simulink model "modelSPSid0"  (R2022a)
settings: Solver=ode45  StartTime=parSimulacio.ti  StopTime=0.1  MaxStep=parSimulacio.pas  RelTol=parSimulacio.tol  EnableMultiTasking=on
undefined symbols (not defined in the file or in its folder): parControl, parConvertidor, parGenerador, parMecanica, parSimulacio
libraries: simulink x7, spsMosfetLib x6, spsCurrentMeasurementLib x4, spsVoltageMeasurementLib x4, spsControlledCurrentSourceLib x3, spsDCVoltageSourceLib x2, spsSeriesRLCBranchLib x2, spspowerguiLib x1
settings Model: SimulationMode=accelerator  Creator=adria  LastModifiedBy=EEED Stores 381
settings SolverCC: AlgebraicLoopSolver=TrustRegion
settings DataIOCC: LimitDataPoints=on  SaveFormat=Array  SignalLoggingSaveFormat=ModelDataLogs  SaveOutput=off  SaveTime=off  ReturnWorkspaceOutputs=off
settings OptimizationCC: InitFltsAndDblsToZero=on  LifeSpan=inf
settings DebuggingCC: SaveWithParameterizedLinksMsg=none  UnderspecifiedInitializationDetection=Classic  MergeDetectMultiDrivingBlocksExec=none  SignalResolutionControl=TryResolveAllWithWarning  SolverPrmCheckMsg=warning  FcnCallInpInsideContextMsg=warning  UnconnectedInputMsg=warning  UnconnectedOutputMsg=warning  UnconnectedLineMsg=warning  SFUnexpectedBacktrackingDiag=warning  SFNoUnconditionalDefaultTransitionDiag=warning  SFExecutionAtInitializationDiag=none  SFMachineParentedDataDiag=warning  ArithmeticOperatorsInVariantConditions=warning
settings HardwareCC: ProdBitPerPointer=32  ProdBitPerSizeT=32  ProdBitPerPtrDiffT=32  ProdLargestAtomicFloat=None  ProdIntDivRoundTo=Undefined  ProdEndianess=Unspecified  ProdWordSize=32  ProdHWDeviceType=32-bit Generic
settings ModelReferenceCC: PropagateSignalLabelsOutOfModel=off
settings RTWCC: DLArmComputeVersion=19.05
settings CodeAppCC: StateflowObjectComments=on
settings GRTTargetCC: TargetFcnLib=ansi_tfl_tmw.mat  TargetLangStandard=C89/C90 (ANSI)  CombineOutputUpdateFcns=off  GRTInterface=on
settings ConfigComp: CovMetricSettings=dw  CovSaveCumulativeToWorkspaceVar=on  CovSaveSingleToWorkspaceVar=on

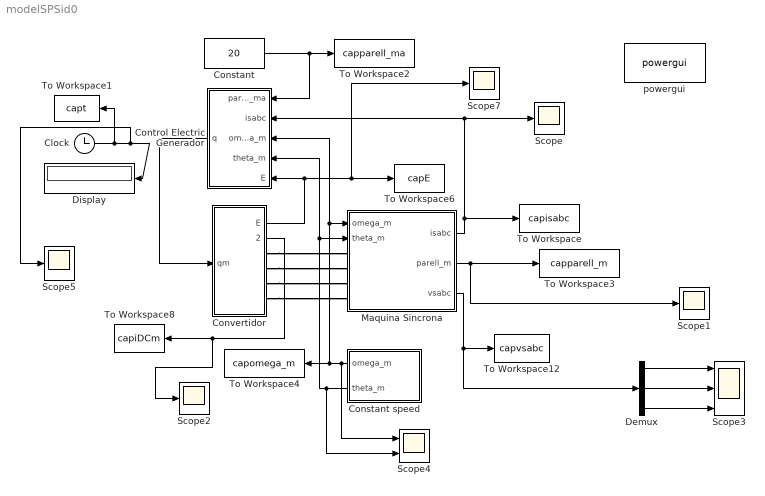
== system modelSPSid0 ==
  Clock : Clock
  Constant : Constant  Value=20
  Constant speed : Subsystem  mask{tempPar=parMecanica}
      mask prompts: tempPar "Estruc. Parametres"
      mask init:
      | omegat0=tempPar.omegat0;
  Control Electric Generador : Subsystem  mask{tempPar=parControl.Electric.Generador}
      mask prompts: tempPar "Estruc. Parametres"
      mask init:
      | rs=tempPar.rs;
      | Lq=tempPar.Lq;
      | Ld=tempPar.Ld;
      | lambda_m=tempPar.lambda_m;
      | P=tempPar.P;
      | %qKp=tempPar.qKp;
      | %qKi=tempPar.qKi;
      | %dKp=tempPar.dKp;
      | %dKi=tempPar.dKi;
      | dGcnum=tempPar.dGcnum;
      | dGcden=tempPar.dGcden;
      | qGcnum=tempPar.qGcnum;
      | qGcden=tempPar.qGcden;
      | T=tempPar.T;
      | SVPWM=tempPar.SVPWM;
  Convertidor : Subsystem  mask{tempPar=parConvertidor}
      mask prompts: tempPar "Estruc. Parametres"
      mask init:
      | E0=tempPar.E0;
      | C=tempPar.C;
  Demux : Demux  Outputs=3
  Display : Display
  Maquina Sincrona : Subsystem  mask{tempPar=parGenerador}
      mask prompts: tempPar "Estruct. Parametres"
      mask init:
      | rs=tempPar.rs;
      | Lq=tempPar.Lq;
      | Ld=tempPar.Ld;
      | lambda_m=tempPar.lambda_m;
      | P=tempPar.P;
      | isqd0=tempPar.isqd0;
  Scope{,1..2,5,7} (5 alike) : Scope
  Scope3 : Scope  NumInputPorts=3
  Scope4 : Scope  NumInputPorts=2
  To Workspace : ToWorkspace  VariableName=capisabc  SampleTime=parSimulacio.captura.Tmostreig
      settings: Decimation=parSimulacio.captura.Delmat
  To Workspace1 : ToWorkspace  VariableName=capt  SampleTime=parSimulacio.captura.Tmostreig
      settings: Decimation=parSimulacio.captura.Delmat
  To Workspace12 : ToWorkspace  VariableName=capvsabc  SampleTime=parSimulacio.captura.Tmostreig
      settings: Decimation=parSimulacio.captura.Delmat
  To Workspace2 : ToWorkspace  VariableName=capparell_ma  SampleTime=parSimulacio.captura.Tmostreig
      settings: Decimation=parSimulacio.captura.Delmat
  To Workspace3 : ToWorkspace  VariableName=capparell_m  SampleTime=parSimulacio.captura.Tmostreig
      settings: Decimation=parSimulacio.captura.Delmat
  To Workspace4 : ToWorkspace  VariableName=capomega_m  SampleTime=parSimulacio.captura.Tmostreig
      settings: Decimation=parSimulacio.captura.Delmat
  To Workspace6 : ToWorkspace  VariableName=capE  SampleTime=parSimulacio.captura.Tmostreig
      settings: Decimation=parSimulacio.captura.Delmat
  To Workspace8 : ToWorkspace  VariableName=capiDCm  SampleTime=parSimulacio.captura.Tmostreig
      settings: Decimation=parSimulacio.captura.Delmat
  powergui : spspowerguiLib/powergui  Priority=1  SimulationMode=Continuous  SampleTime=50e-6  frequency=60  Iterations=50  frequencyindice=0  Pbase=100e6  ErrMax=1e-4  UnitsV=kV  UnitsW=MW  buscounter=0  FunctionMessages=off  echomessages=off  EnableUseOfTLC=off  CurrentSourceSwitches=off  DisableSnubberDevices=off  DisableRonSwitches=off  DisableVfSwitches=off  DisplayEquations=off  AutomaticDiscreteSolvers=off  SolverType=Tustin/Backward Euler (TBE)  Interpol=off  ExternalGateDelay=off  methode=off  Ts=100  x0status=blocks  SPID=on  SwTol=0  HookPort=off  NonlinearTolerance=1e-4  nMaxIteration=100  ContinueOnMaxIteration=off  RestoreLinks=warning  ResistiveCurrentMeasurement=off  Frange=[0:2:500]  Ylog=off  Xlog=on  ShowGrid=off  save=off  variable=ZData  structure=0  ZoomFFT=off  StartTime=0.0  cycles=1  DisplayStyle=1  fundamental=60  FreqAxis=off  MaxFrequency=1000  frequencyindicesteady=1  RmsSteady=1  display=off
  wires:
  Clock/1 -> To Workspace1/1, Scope5/1, Display/1
  Control Electric Generador/1(q) -> Convertidor/1(qm)
  Convertidor/1(E) -> Control Electric Generador/5(E), Scope7/1, To Workspace6/1
  Convertidor/2(iDCm) -> Scope2/1, To Workspace8/1
  Maquina Sincrona/1(isabc) -> Control Electric Generador/2(isabc), Scope/1, To Workspace/1
  Maquina Sincrona/2(parell_m) -> Scope1/1, To Workspace3/1
  Constant speed/1(omega_m) -> Scope4/1, Maquina Sincrona/1(omega_m), Control Electric Generador/3(omega_m), To Workspace4/1
  Constant speed/2(theta_m) -> Scope4/2, Maquina Sincrona/2(theta_m), Control Electric Generador/4(theta_m)
  Maquina Sincrona/3(vsabc) -> To Workspace12/1, Demux/1
  Constant/1 -> Control Electric Generador/1(parell_ma), To Workspace2/1
  Demux/1 -> Scope3/1
  Demux/2 -> Scope3/2
  Demux/3 -> Scope3/3
  connections:
  Convertidor/RConn4 -- Maquina Sincrona/LConn4
  Convertidor/RConn3 -- Maquina Sincrona/LConn3
  Convertidor/RConn2 -- Maquina Sincrona/LConn2
  Convertidor/RConn1 -- Maquina Sincrona/LConn1

== system modelSPSid0/Constant speed ==
  Constant : Constant  Value=omegat0
  Constant1 : Constant  Value=pi/180
  Divide : Product  Inputs=*/  RndMeth=Zero  SaturateOnIntegerOverflow=on
  Divide1 : Product  Inputs=**  RndMeth=Zero  SaturateOnIntegerOverflow=on
  Integrator1 : Integrator
  Round : Rounding  Operator=round
  Scope : Scope  NumInputPorts=2
  Scope1 : Scope  NumInputPorts=2
  omega_m : Outport
  theta_m : Outport  Port=2
  wires:
  Constant/1 -> omega_m/1, Integrator1/1
  Integrator1/1 -> Scope/1, Divide/1
  Constant1/1 -> Divide1/2, Divide/2
  Divide/1 -> Scope1/1, Round/1
  Round/1 -> Scope1/2, Divide1/1
  Divide1/1 -> Scope/2, theta_m/1

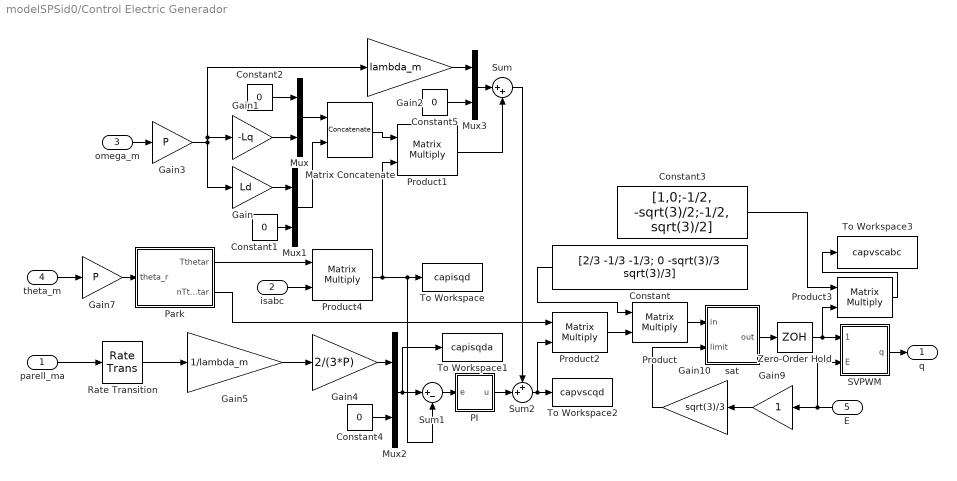
== system modelSPSid0/Control Electric Generador ==
  parell_ma : Inport
  isabc : Inport  Port=2  SampleTime=T
  omega_m : Inport  Port=3  SampleTime=T
  theta_m : Inport  Port=4  PortDimensions=1  SampleTime=T
  E : Inport  Port=5  SampleTime=T
  Constant : Constant  Value=[2/3 -1/3 -1/3; 0 -sqrt(3)/3 sqrt(3)/3]  SampleTime=T
  Constant{1..2,4..5} (4 alike) : Constant  Value=0  SampleTime=T
  Constant3 : Constant  Value=[1,0;-1/2, -sqrt(3)/2;-1/2, sqrt(3)/2]  SampleTime=T
  Gain : Gain  Gain=Ld
  Gain1 : Gain  Gain=-Lq
  Gain10 : Gain  Gain=sqrt(3)/3
  Gain2 : Gain  Gain=lambda_m
  Gain3 : Gain  Gain=P
  Gain4 : Gain  Gain=2/(3*P)
  Gain5 : Gain  Gain=1/lambda_m
  Gain7 : Gain  Gain=P
  Gain9 : Gain  SampleTime=T
  Matrix Concatenate : Concatenate  Mode=Multidimensional array  ConcatenateDimension=2
  Mux{,1..3} (4 alike) : Mux  Inputs=2
  PI : Subsystem
  Park : Subsystem
  Product{,1..4} (5 alike) : Product  Multiplication=Matrix(*)  RndMeth=Zero
  Rate Transition : RateTransition  OutPortSampleTime=T
  SVPWM : Subsystem  mask{TempPar=SVPWM}
      mask prompts: TempPar "Estructura de Parametres"
      mask init:
      | T=TempPar.T;
      | resolucio=TempPar.resolucio;
  Sum : Sum  Inputs=|++
  Sum1 : Sum  Inputs=|+-
  Sum2 : Sum  Inputs=++|
  To Workspace : ToWorkspace  VariableName=capisqd  SampleTime=parSimulacio.captura.Tmostreig
      settings: Decimation=parSimulacio.captura.Delmat
  To Workspace1 : ToWorkspace  VariableName=capisqda  SampleTime=parSimulacio.captura.Tmostreig
      settings: Decimation=parSimulacio.captura.Delmat
  To Workspace2 : ToWorkspace  VariableName=capvscqd  SampleTime=parSimulacio.captura.Tmostreig
      settings: Decimation=parSimulacio.captura.Delmat
  To Workspace3 : ToWorkspace  VariableName=capvscabc  SampleTime=parSimulacio.captura.Tmostreig
      settings: Decimation=parSimulacio.captura.Delmat
  Zero-Order Hold : ZeroOrderHold  SampleTime=T
  sat : Subsystem
  q : Outport
  wires:
  Gain7/1 -> Park/1(theta_r)
  Park/1(Tthetar) -> Product4/1
  Constant2/1 -> Mux/1
  Gain1/1 -> Mux/2
  Gain/1 -> Mux1/1
  Constant1/1 -> Mux1/2
  Mux/1 -> Matrix Concatenate/1
  Mux1/1 -> Matrix Concatenate/2
  Matrix Concatenate/1 -> Product1/1
  Product4/1 -> Product1/2, Sum1/2, To Workspace/1
  omega_m/1 -> Gain3/1
  Product1/1 -> Sum/2
  Sum2/1 -> Product2/2, To Workspace2/1
  Sum1/1 -> PI/1(e)
  PI/1(u) -> Sum2/2
  Mux2/1 -> Sum1/1, To Workspace1/1
  theta_m/1 -> Gain7/1
  isabc/1 -> Product4/2
  Gain3/1 -> Gain1/1, Gain2/1, Gain/1
  Mux3/1 -> Sum/1
  Gain2/1 -> Mux3/1
  Constant5/1 -> Mux3/2
  Park/2(nTthetar) -> Product2/1
  Sum/1 -> Sum2/1
  Gain4/1 -> Mux2/1
  Gain5/1 -> Gain4/1
  parell_ma/1 -> Rate Transition/1
  Rate Transition/1 -> Gain5/1
  Product/1 -> sat/1(in)
  sat/1(out) -> Zero-Order Hold/1
  Gain9/1 -> Gain10/1
  Gain10/1 -> sat/2(limit)
  Zero-Order Hold/1 -> SVPWM/1(valfbet), Product3/2
  E/1 -> Gain9/1, SVPWM/2(E)
  Product2/1 -> Product/2
  Constant/1 -> Product/1
  SVPWM/1(q) -> q/1
  Constant3/1 -> Product3/1
  Product3/1 -> To Workspace3/1
  Constant4/1 -> Mux2/2

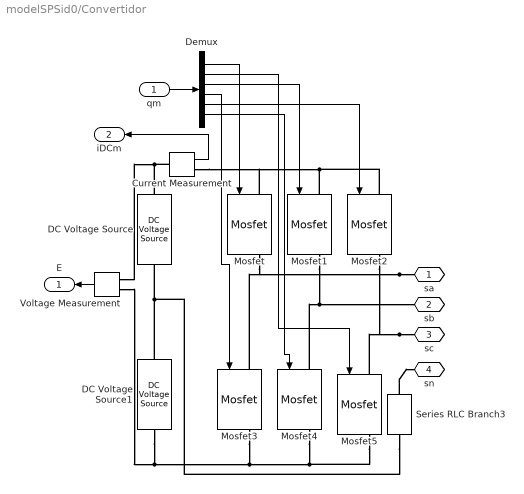
== system modelSPSid0/Convertidor ==
  qm : Inport
  Current Measurement : spsCurrentMeasurementLib/Current Measurement  PhasorSimulation=off  OutputType=Complex  PSBequivalent=0
  DC Voltage Source : spsDCVoltageSourceLib/DC Voltage Source  Amplitude=E0/2  Measurements=None
  DC Voltage Source1 : spsDCVoltageSourceLib/DC Voltage Source  Amplitude=E0/2  Measurements=None
  Demux : Demux  Outputs=6
  Mosfet{,1..5} (6 alike) : spsMosfetLib/Mosfet  Ron=0.1  Lon=0  Rd=0.01  Vfd=0  IC=0  Rs=1e5  Cs=inf  Measurements=on
  Series RLC Branch3 : spsSeriesRLCBranchLib/Series RLC Branch  LConnTagsString=__new0  RConnTagsString=__new0  BranchType=R  Resistance=1e5  Inductance=1e-3  SetiL0=off  InitialCurrent=0  Capacitance=1e-6  Setx0=off  InitialVoltage=0  Measurements=None
  Voltage Measurement : spsVoltageMeasurementLib/Voltage Measurement  PhasorSimulation=off  OutputType=Complex  PSBequivalent=0
  sa : PMIOPort  Side=Right
  sb : PMIOPort  Port=2  Side=Right
  sc : PMIOPort  Port=3  Side=Right
  sn : PMIOPort  Port=4  Side=Right
  E : Outport
  iDCm : Outport  Port=2
  wires:
  Voltage Measurement/1 -> E/1
  Demux/1 -> Mosfet/1
  Demux/3 -> Mosfet1/1
  Demux/5 -> Mosfet2/1
  Demux/2 -> Mosfet5/1
  Demux/4 -> Mosfet3/1
  Demux/6 -> Mosfet4/1
  qm/1 -> Demux/1
  Current Measurement/1 -> iDCm/1
  connections:
  sa/RConn1 -- Mosfet3/LConn1 -- Mosfet/RConn1
  Mosfet1/RConn1 -- Mosfet4/LConn1 -- sb/RConn1
  sc/RConn1 -- Mosfet5/LConn1 -- Mosfet2/RConn1
  Mosfet/LConn1 -- Current Measurement/RConn1 -- Mosfet2/LConn1 -- Mosfet1/LConn1
  Series RLC Branch3/RConn1 -- sn/RConn1
  DC Voltage Source1/RConn1 -- Series RLC Branch3/LConn1 -- DC Voltage Source/LConn1
  DC Voltage Source/RConn1 -- Voltage Measurement/LConn1 -- Current Measurement/LConn1
  DC Voltage Source1/LConn1 -- Voltage Measurement/LConn2 -- Mosfet3/RConn1 -- Mosfet5/RConn1 -- Mosfet4/RConn1

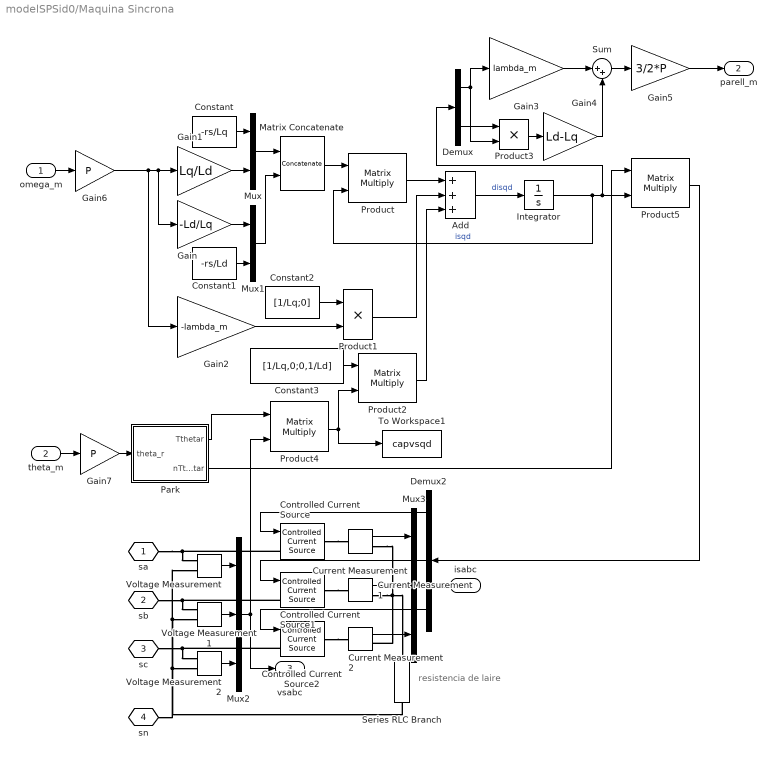
== system modelSPSid0/Maquina Sincrona ==
  note: resistencia
      | de laire
  omega_m : Inport
  theta_m : Inport  Port=2  PortDimensions=1
  Add : Sum  Inputs=+++
  Constant : Constant  Value=-rs/Lq
  Constant1 : Constant  Value=-rs/Ld
  Constant2 : Constant  Value=[1/Lq;0]
  Constant3 : Constant  Value=[1/Lq,0;0,1/Ld]
  Controlled Current Source : spsControlledCurrentSourceLib/Controlled Current Source  Initialize=on  Source_Type=AC  Amplitude=0  Phase=0  Frequency=0  Measurements=None
  Controlled Current Source1 : spsControlledCurrentSourceLib/Controlled Current Source  Initialize=on  Source_Type=AC  Amplitude=0  Phase=0  Frequency=0  Measurements=None
  Controlled Current Source2 : spsControlledCurrentSourceLib/Controlled Current Source  Initialize=on  Source_Type=AC  Amplitude=0  Phase=0  Frequency=0  Measurements=None
  Current Measurement : spsCurrentMeasurementLib/Current Measurement  PhasorSimulation=off  OutputType=Complex  PSBequivalent=0
  Current Measurement1 : spsCurrentMeasurementLib/Current Measurement  PhasorSimulation=off  OutputType=Complex  PSBequivalent=0
  Current Measurement2 : spsCurrentMeasurementLib/Current Measurement  PhasorSimulation=off  OutputType=Complex  PSBequivalent=0
  Demux : Demux  Outputs=2
  Demux2 : Demux  Outputs=3
  Gain : Gain  Gain=-Ld/Lq
  Gain1 : Gain  Gain=Lq/Ld
  Gain2 : Gain  Gain=-lambda_m
  Gain3 : Gain  Gain=lambda_m
  Gain4 : Gain  Gain=Ld-Lq
  Gain5 : Gain  Gain=3/2*P
  Gain6 : Gain  Gain=P
  Gain7 : Gain  Gain=P
  Integrator : Integrator  InitialCondition=isqd0
  Matrix Concatenate : Concatenate  Mode=Multidimensional array  ConcatenateDimension=2
  Mux : Mux  Inputs=2
  Mux1 : Mux  Inputs=2
  Mux2 : Mux  Inputs=3
  Mux3 : Mux  Inputs=3
  Park : Subsystem
  Product{,2,4..5} (4 alike) : Product  Multiplication=Matrix(*)  RndMeth=Zero
  Product1 : Product  RndMeth=Zero
  Product3 : Product  RndMeth=Zero
  Series RLC Branch : spsSeriesRLCBranchLib/Series RLC Branch  LConnTagsString=__new0  RConnTagsString=__new0  BranchType=R  Resistance=1e5  Inductance=1e-3  SetiL0=off  InitialCurrent=0  Capacitance=1e-6  Setx0=off  InitialVoltage=0  Measurements=None
  Sum : Sum  Inputs=|++
  To Workspace1 : ToWorkspace  VariableName=capvsqd  SampleTime=parSimulacio.captura.Tmostreig
      settings: Decimation=parSimulacio.captura.Delmat
  Voltage Measurement : spsVoltageMeasurementLib/Voltage Measurement  PhasorSimulation=off  OutputType=Complex  PSBequivalent=0
  Voltage Measurement1 : spsVoltageMeasurementLib/Voltage Measurement  PhasorSimulation=off  OutputType=Complex  PSBequivalent=0
  Voltage Measurement2 : spsVoltageMeasurementLib/Voltage Measurement  PhasorSimulation=off  OutputType=Complex  PSBequivalent=0
  sa : PMIOPort  Tag=PMCPort  Side=Left
  sb : PMIOPort  Tag=PMCPort  Port=2  Side=Left
  sc : PMIOPort  Tag=PMCPort  Port=3  Side=Left
  sn : PMIOPort  Tag=PMCPort  Port=4  Side=Left
  isabc : Outport
  parell_m : Outport  Port=2
  vsabc : Outport  Port=3
  wires:
  Constant/1 -> Mux/1
  Gain1/1 -> Mux/2
  Gain/1 -> Mux1/1
  Constant1/1 -> Mux1/2
  omega_m/1 -> Gain6/1
  Mux/1 -> Matrix Concatenate/1
  Mux1/1 -> Matrix Concatenate/2
  Matrix Concatenate/1 -> Product/1
  Product/1 -> Add/1
  Add/1 -> Integrator/1  "disqd"
  Integrator/1 -> Demux/1, Product5/2, Product/2  "isqd"
  Gain2/1 -> Product1/2
  Constant2/1 -> Product1/1
  Product1/1 -> Add/2
  Constant3/1 -> Product2/1
  Product2/1 -> Add/3
  Demux/1 -> Gain3/1, Product3/2
  Product3/1 -> Gain4/1
  Demux/2 -> Product3/1
  Gain3/1 -> Sum/1
  Gain4/1 -> Sum/2
  Sum/1 -> Gain5/1
  Gain5/1 -> parell_m/1
  Gain6/1 -> Gain1/1, Gain/1, Gain2/1
  theta_m/1 -> Gain7/1
  Product4/1 -> Product2/2, To Workspace1/1
  Park/1(Tthetar) -> Product4/1
  Gain7/1 -> Park/1(theta_r)
  Park/2(nTthetar) -> Product5/1
  Demux2/1 -> Controlled Current Source/1
  Demux2/2 -> Controlled Current Source1/1
  Demux2/3 -> Controlled Current Source2/1
  Voltage Measurement/1 -> Mux2/1
  Voltage Measurement1/1 -> Mux2/2
  Voltage Measurement2/1 -> Mux2/3
  Current Measurement/1 -> Mux3/1
  Current Measurement2/1 -> Mux3/3
  Product5/1 -> Demux2/1
  Current Measurement1/1 -> Mux3/2
  Mux3/1 -> isabc/1
  Mux2/1 -> Product4/2, vsabc/1
  connections:
  Controlled Current Source2/RConn1 -- Current Measurement2/LConn1
  Controlled Current Source1/RConn1 -- Current Measurement1/LConn1
  Controlled Current Source/RConn1 -- Current Measurement/LConn1
  Current Measurement/RConn1 -- Current Measurement2/RConn1 -- Current Measurement1/RConn1 -- Series RLC Branch/LConn1
  Controlled Current Source1/LConn1 -- Voltage Measurement1/LConn1 -- sb/RConn1
  Controlled Current Source2/LConn1 -- Voltage Measurement2/LConn1 -- sc/RConn1
  Controlled Current Source/LConn1 -- Voltage Measurement/LConn1 -- sa/RConn1
  sn/RConn1 -- Series RLC Branch/RConn1 -- Voltage Measurement2/LConn2 -- Voltage Measurement1/LConn2 -- Voltage Measurement/LConn2

== system modelSPSid0/Control Electric Generador/PI ==
  e : Inport
  Demux : Demux  Outputs=2
  Discrete Transfer Fcn : DiscreteTransferFcn  Numerator=[qGcnum]  Denominator=[qGcden]  SampleTime=T
  Discrete Transfer Fcn1 : DiscreteTransferFcn  Numerator=[dGcnum]  Denominator=[dGcden]  SampleTime=T
  Mux2 : Mux  Inputs=2
  u : Outport
  wires:
  Discrete Transfer Fcn/1 -> Mux2/1
  Discrete Transfer Fcn1/1 -> Mux2/2
  Demux/1 -> Discrete Transfer Fcn/1
  Demux/2 -> Discrete Transfer Fcn1/1
  e/1 -> Demux/1
  Mux2/1 -> u/1

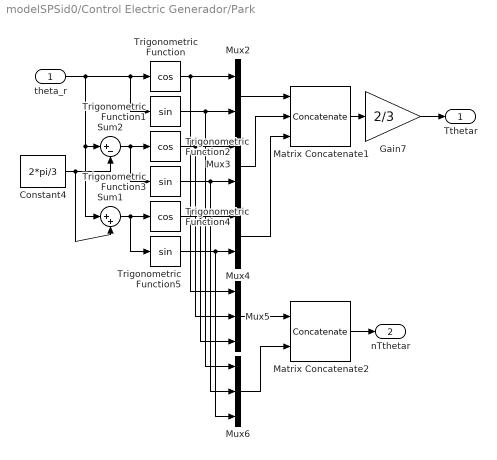
== system modelSPSid0/Control Electric Generador/Park ==
  theta_r : Inport
  Constant4 : Constant  Value=2*pi/3  SampleTime=T
  Gain7 : Gain  Gain=2/3
  Matrix Concatenate1 : Concatenate  NumInputs=3  Mode=Multidimensional array  ConcatenateDimension=2
  Matrix Concatenate2 : Concatenate  Mode=Multidimensional array  ConcatenateDimension=2
  Mux2 : Mux  Inputs=2
  Mux3 : Mux  Inputs=2
  Mux4 : Mux  Inputs=2
  Mux5 : Mux  Inputs=3
  Mux6 : Mux  Inputs=3
  Sum1 : Sum  Inputs=|++
  Sum2 : Sum  Inputs=|+-
  Trigonometric Function : Trigonometry  Operator=cos
  Trigonometric Function1 : Trigonometry
  Trigonometric Function2 : Trigonometry  Operator=cos
  Trigonometric Function3 : Trigonometry
  Trigonometric Function4 : Trigonometry  Operator=cos
  Trigonometric Function5 : Trigonometry
  Tthetar : Outport
  nTthetar : Outport  Port=2
  wires:
  theta_r/1 -> Sum1/1, Sum2/1, Trigonometric Function/1, Trigonometric Function1/1
  Sum2/1 -> Trigonometric Function2/1, Trigonometric Function3/1
  Sum1/1 -> Trigonometric Function4/1, Trigonometric Function5/1
  Constant4/1 -> Sum2/2, Sum1/2
  Trigonometric Function/1 -> Mux2/1, Mux5/1
  Trigonometric Function1/1 -> Mux2/2, Mux6/1
  Trigonometric Function2/1 -> Mux3/1, Mux5/2
  Trigonometric Function3/1 -> Mux3/2, Mux6/2
  Trigonometric Function4/1 -> Mux4/1, Mux5/3
  Trigonometric Function5/1 -> Mux4/2, Mux6/3
  Mux2/1 -> Matrix Concatenate1/1
  Mux3/1 -> Matrix Concatenate1/2
  Mux4/1 -> Matrix Concatenate1/3
  Matrix Concatenate1/1 -> Gain7/1
  Mux5/1 -> Matrix Concatenate2/1
  Mux6/1 -> Matrix Concatenate2/2
  Gain7/1 -> Tthetar/1
  Matrix Concatenate2/1 -> nTthetar/1

== system modelSPSid0/Control Electric Generador/SVPWM ==
  valfbet : Inport
  E : Inport  Port=2
  Calcul Periodes : Subsystem
  Dispars : Subsystem
  Divide1 : Product  Inputs=*/
  Gain1 : Gain  SampleTime=T
  Gain10 : Gain  Gain=sqrt(3)/3
  Mux : Mux  Inputs=6
  Rate Transition1 : RateTransition  OutPortSampleTime=T
  sat : Subsystem
  q : Outport
  wires:
  valfbet/1 -> Rate Transition1/1
  Calcul Periodes/1(t) -> Dispars/1(t)
  Calcul Periodes/2(n) -> Dispars/2(n)
  E/1 -> Gain1/1
  Rate Transition1/1 -> sat/1(in)
  Gain10/1 -> sat/2(limit)
  Divide1/1 -> Calcul Periodes/1(vsc)
  sat/1(out) -> Divide1/1
  Gain1/1 -> Gain10/1, Divide1/2
  Dispars/1(q1) -> Mux/1
  Dispars/2(q2) -> Mux/2
  Dispars/3(q3) -> Mux/3
  Dispars/4(q4) -> Mux/4
  Dispars/5(q5) -> Mux/5
  Dispars/6(q6) -> Mux/6
  Mux/1 -> q/1

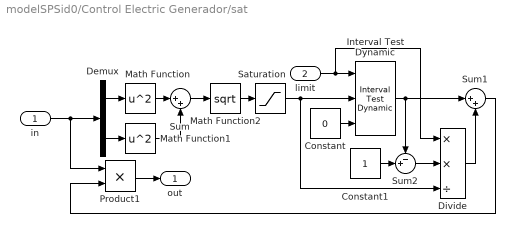
== system modelSPSid0/Control Electric Generador/sat ==
  in : Inport
  limit : Inport  Port=2
  Constant : Constant  Value=0  SampleTime=T
  Constant1 : Constant  SampleTime=T
  Demux : Demux  Outputs=2
  Divide : Product  Inputs=**/
  Interval Test Dynamic : simulink/Logic and Bit Operations/Interval Test Dynamic  IntervalClosedRight=on  IntervalClosedLeft=on  OutDataTypeStr=uint8
      settings: SourceProductBaseCode=SL
  Math Function : Math  Operator=square  SignedPower=on
  Math Function1 : Math  Operator=square  SignedPower=on
  Math Function2 : Math  Operator=sqrt  SignedPower=on
  Product1 : Product  RndMeth=Zero
  Saturation : Saturate  UpperLimit=inf  LowerLimit=1
  Sum : Sum  Inputs=|++
  Sum1 : Sum  Inputs=|++
  Sum2 : Sum  Inputs=-+|
  out : Outport
  wires:
  Math Function/1 -> Sum/1
  Math Function1/1 -> Sum/2
  Sum/1 -> Math Function2/1
  Math Function2/1 -> Saturation/1
  Demux/1 -> Math Function/1
  Demux/2 -> Math Function1/1
  in/1 -> Demux/1, Product1/1
  Product1/1 -> out/1
  Constant/1 -> Interval Test Dynamic/3
  Interval Test Dynamic/1 -> Sum1/1, Sum2/1
  Constant1/1 -> Sum2/2
  limit/1 -> Divide/1, Interval Test Dynamic/1
  Sum2/1 -> Divide/2
  Divide/1 -> Sum1/2
  Sum1/1 -> Product1/2
  Saturation/1 -> Divide/3, Interval Test Dynamic/2

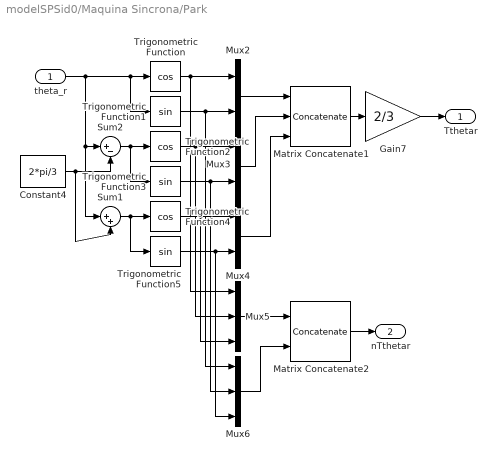
== system modelSPSid0/Maquina Sincrona/Park ==
  theta_r : Inport
  Constant4 : Constant  Value=2*pi/3
  Gain7 : Gain  Gain=2/3
  Matrix Concatenate1 : Concatenate  NumInputs=3  Mode=Multidimensional array  ConcatenateDimension=2
  Matrix Concatenate2 : Concatenate  Mode=Multidimensional array  ConcatenateDimension=2
  Mux2 : Mux  Inputs=2
  Mux3 : Mux  Inputs=2
  Mux4 : Mux  Inputs=2
  Mux5 : Mux  Inputs=3
  Mux6 : Mux  Inputs=3
  Sum1 : Sum  Inputs=|++
  Sum2 : Sum  Inputs=|+-
  Trigonometric Function : Trigonometry  Operator=cos
  Trigonometric Function1 : Trigonometry
  Trigonometric Function2 : Trigonometry  Operator=cos
  Trigonometric Function3 : Trigonometry
  Trigonometric Function4 : Trigonometry  Operator=cos
  Trigonometric Function5 : Trigonometry
  Tthetar : Outport
  nTthetar : Outport  Port=2
  wires:
  theta_r/1 -> Sum1/1, Sum2/1, Trigonometric Function/1, Trigonometric Function1/1
  Sum2/1 -> Trigonometric Function2/1, Trigonometric Function3/1
  Sum1/1 -> Trigonometric Function4/1, Trigonometric Function5/1
  Constant4/1 -> Sum2/2, Sum1/2
  Trigonometric Function/1 -> Mux2/1, Mux5/1
  Trigonometric Function1/1 -> Mux2/2, Mux6/1
  Trigonometric Function2/1 -> Mux3/1, Mux5/2
  Trigonometric Function3/1 -> Mux3/2, Mux6/2
  Trigonometric Function4/1 -> Mux4/1, Mux5/3
  Trigonometric Function5/1 -> Mux4/2, Mux6/3
  Mux2/1 -> Matrix Concatenate1/1
  Mux3/1 -> Matrix Concatenate1/2
  Mux4/1 -> Matrix Concatenate1/3
  Matrix Concatenate1/1 -> Gain7/1
  Mux5/1 -> Matrix Concatenate2/1
  Mux6/1 -> Matrix Concatenate2/2
  Gain7/1 -> Tthetar/1
  Matrix Concatenate2/1 -> nTthetar/1

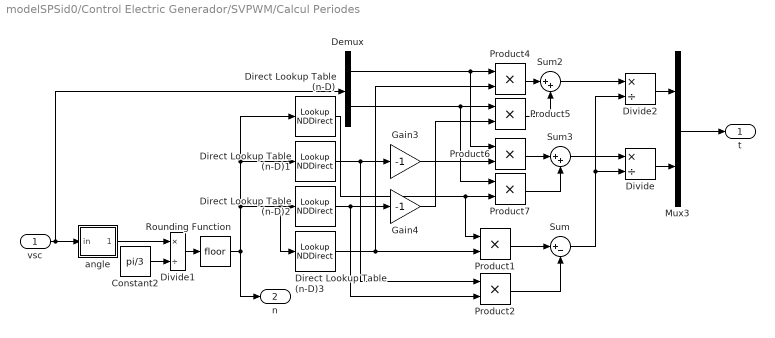
== system modelSPSid0/Control Electric Generador/SVPWM/Calcul Periodes ==
  vsc : Inport
  Constant2 : Constant  Value=pi/3  SampleTime=T
  Demux : Demux  Outputs=2
  Direct Lookup Table (n-D) : LookupNDDirect  NumberOfTableDimensions=1  Table=[2/3, 1/3, -1/3, -2/3, -1/3, 1/3]
  Direct Lookup Table (n-D)1 : LookupNDDirect  NumberOfTableDimensions=1  Table=[0, -sqrt(3)/3, -sqrt(3)/3, 0 ,sqrt(3)/3, sqrt(3)/3]
  Direct Lookup Table (n-D)2 : LookupNDDirect  NumberOfTableDimensions=1  Table=[1/3, -1/3, -2/3, -1/3, 1/3,2/3]
  Direct Lookup Table (n-D)3 : LookupNDDirect  NumberOfTableDimensions=1  Table=[-sqrt(3)/3, -sqrt(3)/3, 0 ,sqrt(3)/3, sqrt(3)/3,0]
  Divide : Product  Inputs=*/
  Divide1 : Product  Inputs=*/
  Divide2 : Product  Inputs=*/
  Gain3 : Gain  Gain=-1
  Gain4 : Gain  Gain=-1
  Mux3 : Mux  Inputs=2
  Product{1..2,4..7} (6 alike) : Product  RndMeth=Zero
  Rounding Function : Rounding
  Sum : Sum  Inputs=|+-
  Sum2 : Sum  Inputs=|++
  Sum3 : Sum  Inputs=|++
  angle : Subsystem
  t : Outport
  n : Outport  Port=2
  wires:
  angle/1(out) -> Divide1/1
  Constant2/1 -> Divide1/2
  Divide1/1 -> Rounding Function/1
  Rounding Function/1 -> n/1, Direct Lookup Table (n-D)1/1, Direct Lookup Table (n-D)/1, Direct Lookup Table (n-D)3/1, Direct Lookup Table (n-D)2/1
  vsc/1 -> angle/1(in), Demux/1
  Product1/1 -> Sum/1
  Product2/1 -> Sum/2
  Sum/1 -> Divide/2, Divide2/2
  Divide2/1 -> Mux3/1
  Divide/1 -> Mux3/2
  Mux3/1 -> t/1
  Product4/1 -> Sum2/1
  Product7/1 -> Sum3/2
  Sum3/1 -> Divide/1
  Sum2/1 -> Divide2/1
  Demux/1 -> Product4/1, Product6/1
  Demux/2 -> Product5/1, Product7/1
  Direct Lookup Table (n-D)3/1 -> Product4/2, Product1/2
  Direct Lookup Table (n-D)2/1 -> Product2/2, Gain4/1
  Gain4/1 -> Product5/2
  Direct Lookup Table (n-D)1/1 -> Gain3/1, Product2/1
  Gain3/1 -> Product6/2
  Direct Lookup Table (n-D)/1 -> Product7/2, Product1/1
  Product5/1 -> Sum2/2
  Product6/1 -> Sum3/1

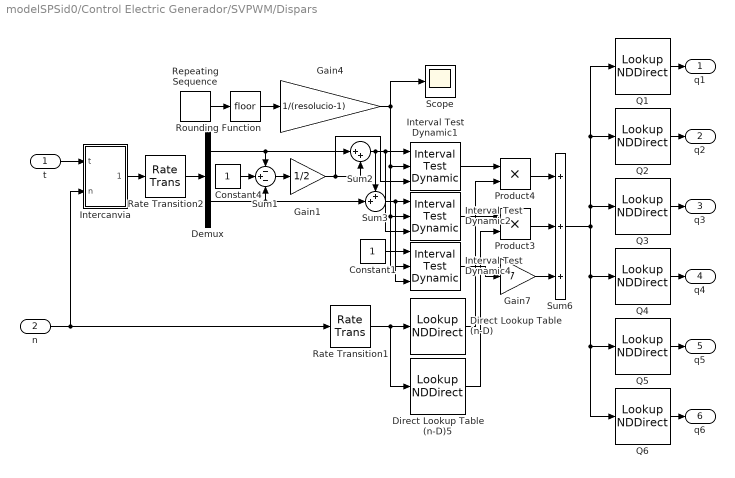
== system modelSPSid0/Control Electric Generador/SVPWM/Dispars ==
  t : Inport
  n : Inport  Port=2
  Constant1 : Constant  SampleTime=T/resolucio
  Constant4 : Constant  SampleTime=T/resolucio
  Demux : Demux  Outputs=2
  Direct Lookup Table (n-D) : LookupNDDirect  NumberOfTableDimensions=1  Table=[1,3,3,5,5,1]
  Direct Lookup Table (n-D)5 : LookupNDDirect  NumberOfTableDimensions=1  Table=[2,2,4,4,6,6]
  Gain1 : Gain  Gain=1/2  SampleTime=parControl.Electric.Generador.T/64
  Gain4 : Gain  Gain=1/(resolucio-1)  SampleTime=T/resolucio
  Gain7 : Gain  Gain=7
  Intercanvia : Subsystem
  Interval Test Dynamic1 : simulink/Logic and Bit Operations/Interval Test Dynamic  IntervalClosedRight=off  IntervalClosedLeft=on  OutDataTypeStr=uint8
      settings: SourceProductBaseCode=SL
  Interval Test Dynamic2 : simulink/Logic and Bit Operations/Interval Test Dynamic  IntervalClosedRight=off  IntervalClosedLeft=on  OutDataTypeStr=uint8
      settings: SourceProductBaseCode=SL
  Interval Test Dynamic4 : simulink/Logic and Bit Operations/Interval Test Dynamic  IntervalClosedRight=on  IntervalClosedLeft=on  OutDataTypeStr=uint8
      settings: SourceProductBaseCode=SL
  Product3 : Product  RndMeth=Zero
  Product4 : Product  RndMeth=Zero
  Q1 : LookupNDDirect  NumberOfTableDimensions=1  Table=[0,1,1,0,0,0,1,1]
  Q2 : LookupNDDirect  NumberOfTableDimensions=1  Table=[1,1,1,1,0,0,0,0]
  Q3 : LookupNDDirect  NumberOfTableDimensions=1  Table=[0,0,1,1,1,0,0,1]
  Q4 : LookupNDDirect  NumberOfTableDimensions=1  Table=[1,0,0,1,1,1,0,0]
  Q5 : LookupNDDirect  NumberOfTableDimensions=1  Table=[0,0,0,0,1,1,1,1]
  Q6 : LookupNDDirect  NumberOfTableDimensions=1  Table=[1,1,0,0,0,1,1,0]
  Rate Transition1 : RateTransition  OutPortSampleTime=T/resolucio
  Rate Transition2 : RateTransition  OutPortSampleTime=T/resolucio
  Repeating Sequence : simulink/Sources/Repeating Sequence  rep_seq_t=[0, T, 2*T]  rep_seq_y=[0,resolucio-1e-3,0]
  Rounding Function : Rounding
  Scope : Scope
  Sum1 : Sum  Inputs=-+-
  Sum2 : Sum  Inputs=|++
  Sum3 : Sum  Inputs=++|
  Sum6 : Sum  Inputs=+++
  q1 : Outport
  q2 : Outport  Port=2
  q3 : Outport  Port=3
  q4 : Outport  Port=4
  q5 : Outport  Port=5
  q6 : Outport  Port=6
  wires:
  Interval Test Dynamic1/1 -> Product4/1
  Interval Test Dynamic2/1 -> Product3/1
  Repeating Sequence/1 -> Rounding Function/1
  Gain4/1 -> Interval Test Dynamic1/2, Interval Test Dynamic2/2, Interval Test Dynamic4/2, Scope/1
  Constant4/1 -> Sum1/2
  Demux/1 -> Sum1/1, Sum2/1
  Demux/2 -> Sum1/3, Sum3/2
  Sum1/1 -> Gain1/1
  Gain1/1 -> Sum2/2, Interval Test Dynamic1/3
  Sum2/1 -> Sum3/1, Interval Test Dynamic1/1, Interval Test Dynamic2/3
  Sum3/1 -> Interval Test Dynamic2/1, Interval Test Dynamic4/3
  Constant1/1 -> Interval Test Dynamic4/1
  Product4/1 -> Sum6/1
  Product3/1 -> Sum6/2
  Gain7/1 -> Sum6/3
  Direct Lookup Table (n-D)/1 -> Product4/2
  Direct Lookup Table (n-D)5/1 -> Product3/2
  Sum6/1 -> Q1/1, Q2/1, Q3/1, Q4/1, Q5/1, Q6/1
  Q1/1 -> q1/1
  Q2/1 -> q2/1
  Q3/1 -> q3/1
  Q4/1 -> q4/1
  Q5/1 -> q5/1
  Q6/1 -> q6/1
  Rate Transition2/1 -> Demux/1
  Rounding Function/1 -> Gain4/1
  t/1 -> Intercanvia/1(t)
  Interval Test Dynamic4/1 -> Gain7/1
  n/1 -> Intercanvia/2(n), Rate Transition1/1
  Intercanvia/1(tswap) -> Rate Transition2/1
  Rate Transition1/1 -> Direct Lookup Table (n-D)/1, Direct Lookup Table (n-D)5/1

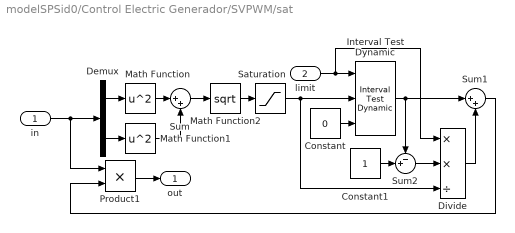
== system modelSPSid0/Control Electric Generador/SVPWM/sat ==
  in : Inport
  limit : Inport  Port=2
  Constant : Constant  Value=0  SampleTime=T
  Constant1 : Constant  SampleTime=T
  Demux : Demux  Outputs=2
  Divide : Product  Inputs=**/
  Interval Test Dynamic : simulink/Logic and Bit Operations/Interval Test Dynamic  IntervalClosedRight=on  IntervalClosedLeft=on  OutDataTypeStr=uint8
      settings: SourceProductBaseCode=SL
  Math Function : Math  Operator=square  SignedPower=on
  Math Function1 : Math  Operator=square  SignedPower=on
  Math Function2 : Math  Operator=sqrt  SignedPower=on
  Product1 : Product  RndMeth=Zero
  Saturation : Saturate  UpperLimit=inf  LowerLimit=1
  Sum : Sum  Inputs=|++
  Sum1 : Sum  Inputs=|++
  Sum2 : Sum  Inputs=-+|
  out : Outport
  wires:
  Math Function/1 -> Sum/1
  Math Function1/1 -> Sum/2
  Sum/1 -> Math Function2/1
  Math Function2/1 -> Saturation/1
  Demux/1 -> Math Function/1
  Demux/2 -> Math Function1/1
  in/1 -> Demux/1, Product1/1
  Product1/1 -> out/1
  Constant/1 -> Interval Test Dynamic/3
  Interval Test Dynamic/1 -> Sum1/1, Sum2/1
  Constant1/1 -> Sum2/2
  limit/1 -> Divide/1, Interval Test Dynamic/1
  Sum2/1 -> Divide/2
  Divide/1 -> Sum1/2
  Sum1/1 -> Product1/2
  Saturation/1 -> Divide/3, Interval Test Dynamic/2

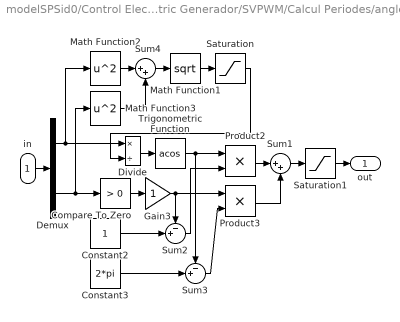
== system modelSPSid0/Control Electric Generador/SVPWM/Calcul Periodes/angle ==
  in : Inport
  Compare To Zero : simulink/Logic and Bit Operations/Compare To Zero  relop=>  OutDataTypeStr=uint8  ZeroCross=off
  Constant2 : Constant  SampleTime=T
  Constant3 : Constant  Value=2*pi  SampleTime=T
  Demux : Demux  Outputs=2
  Divide : Product  Inputs=*/
  Gain3 : Gain  SampleTime=T
  Math Function1 : Math  Operator=sqrt  SignedPower=on
  Math Function2 : Math  Operator=square  SignedPower=on
  Math Function3 : Math  Operator=square  SignedPower=on
  Product2 : Product  RndMeth=Zero
  Product3 : Product  RndMeth=Zero
  Saturation : Saturate  UpperLimit=inf  LowerLimit=1e-3
  Saturation1 : Saturate  UpperLimit=2*pi-1e-3  LowerLimit=0
  Sum1 : Sum  Inputs=|++
  Sum2 : Sum  Inputs=-+|
  Sum3 : Sum  Inputs=-+|
  Sum4 : Sum  Inputs=|++
  Trigonometric Function : Trigonometry  Operator=acos
  out : Outport
  wires:
  Demux/2 -> Compare To Zero/1, Math Function3/1
  Constant2/1 -> Sum2/2
  Compare To Zero/1 -> Gain3/1
  Trigonometric Function/1 -> Sum3/1, Product2/1
  Sum2/1 -> Product2/2
  Constant3/1 -> Sum3/2
  Sum3/1 -> Product3/2
  Product2/1 -> Sum1/1
  Product3/1 -> Sum1/2
  in/1 -> Demux/1
  Sum1/1 -> Saturation1/1
  Gain3/1 -> Sum2/1, Product3/1
  Divide/1 -> Trigonometric Function/1
  Demux/1 -> Math Function2/1, Divide/1
  Math Function2/1 -> Sum4/1
  Math Function3/1 -> Sum4/2
  Sum4/1 -> Math Function1/1
  Math Function1/1 -> Saturation/1
  Saturation/1 -> Divide/2
  Saturation1/1 -> out/1

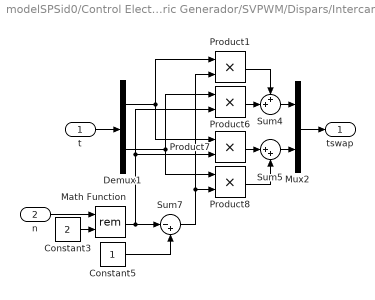
== system modelSPSid0/Control Electric Generador/SVPWM/Dispars/Intercanvia ==
  t : Inport
  n : Inport  Port=2
  Constant3 : Constant  Value=2  SampleTime=parControl.Electric.Generador.T/64
  Constant5 : Constant  SampleTime=parControl.Electric.Generador.T/64
  Demux1 : Demux  Outputs=2
  Math Function : Math  Operator=rem  SignedPower=on
  Mux2 : Mux  Inputs=2
  Product{1,6..8} (4 alike) : Product  RndMeth=Zero
  Sum4 : Sum  Inputs=++|
  Sum5 : Sum  Inputs=|++
  Sum7 : Sum  Inputs=|-+
  tswap : Outport
  wires:
  Sum4/1 -> Mux2/1
  Sum5/1 -> Mux2/2
  Product1/1 -> Sum4/1
  Product6/1 -> Sum4/2
  Product7/1 -> Sum5/1
  Product8/1 -> Sum5/2
  Demux1/1 -> Product1/1, Product7/1
  Demux1/2 -> Product6/1, Product8/1
  Constant3/1 -> Math Function/2
  Math Function/1 -> Sum7/1, Product6/2, Product7/2
  Constant5/1 -> Sum7/2
  n/1 -> Math Function/1
  t/1 -> Demux1/1
  Mux2/1 -> tswap/1
  Sum7/1 -> Product1/2, Product8/2
